simulink library "tp333079"  (Simulink 5.0)
values from neighbouring files (symbols this model uses):
  b = 1    [main_flock3.m]    (also in main_flock4.m; params_flocking_ros.m)
undefined symbols (not defined in the file or in its folder): AC, AlphaBnd, BetaBnd, CDda, CDde, CDdf, CDdr, CDM, CDmin, CGempty, CGgross, CL0, CLa, CLalphadot, Clbeta, Clda, CLde, CLdf, Cldr, CLM, CLmind, Clp, CLq, Clr, Cm0, Cma, Cmalphadot, Cmde, Cmdf, CmM, Cmq, Cnbeta, Cnda, Cndr, Cnp, Cnr, CP, CT, CYbeta, CYda, CYdr, CYp, CYr, Displacement, dmy, Engine, EulerIni, FuelFlow, FuelIni, J, Jempty, Jeng, Jgross, Jprop, MAC, MAP, MAPLim, MassIni, MaxPower, mempty ... (+26)
libraries: aerosimlib x325, simulink3 x42
(part 2 of 11)

== system tp333079/Inertia ==
  Aircraft Inertia : Subsystem  SimViewingDevice=off  mask(Aircraft inertia){FuelIni=FuelIni, Mempty=mempty, Mgross=mgross, CGempty=CGempty, CGgross=CGgross, Jempty=Jempty, Jgross=Jgross}
      mask prompts: FuelIni "Initial fuel mass:"; Mempty "Empty mass:"; Mgross "Gross mass:"; CGempty "Empty CG location [X Y Z]:"; CGgross "Gross CG location [X Y Z]:"; Jempty "Empty moments of inertia [Jx Jy Jz Jxz]:"; Jgross "Gross moments of inertia [Jx Jy Jz Jxz]:"
      mask help: Computes the current aircraft inertia parameters (mass, CG location and moments of inertia) given the fuel flow.
      settings: Permissions=ReadWrite  RTWFcnNameOpts=Auto  RTWFileNameOpts=Auto
      mask Help:
      | The block integrates the fuel flow rate and updates the inertia parameters of the airpane knowing the current fuel quantity.
      | <P><B>Parameters:</B>
      | <LI>Initial fuel mass;</LI>
      | <LI>Mass of empty aircraft;</LI>
      | <LI>Gross mass of the aircraft;</LI>
      | <LI>The 3x1 position vector from origin to the empty aircraft CG location;</LI>
      | <LI>The 3x1 position vector from origin to the gross aircraft CG location;</LI>
      | <LI>The 4x1 vector of moments of inertia for the empty aircraft;</LI>
      | <LI>The 4x1 vector of moments of inertia for the gross aircraft;</LI>
      | </P>
      | <P><B>Inputs:</B>
      | <LI>Fuel flow;</LI>
      | <LI>Reset flag, for resetting the fuel integrator back to the initial value;</LI>
      | </P>
      | <P><B>Outputs:</B>
      | <LI>Current aircraft mass;</LI>
      | <LI>Current aircraft CG location;</LI>
      | <LI>Current aircraft moments of inertia.</LI>
      | <LI>Flag that gets set to 1 if the aircraft is out of fuel.</LI>
      | </P>
  Inertia Coefficients : Subsystem  SimViewingDevice=off
      settings: Permissions=ReadWrite  RTWFcnNameOpts=Auto  RTWFileNameOpts=Auto
      mask Type: Inertia coefficients
      mask Description: Compute inertia coefficients c1-c10 based on moments of inertia.
      mask Help:
      | The block computes the coefficients c1-c10 which are elements of the inverse of the moments of inertia matrix, used in the rigid body moment equations.
      | <P><B>Input:</B> 4x1 vector of moments of inertia;</P>
      | <P><B>Output:</B> 10x1 vector of inertia coefficients.</P>

== system tp333079/Math ==
  2pi Bound : Subsystem  SimViewingDevice=off
      settings: Permissions=ReadWrite  RTWFcnNameOpts=Auto  RTWFileNameOpts=Auto
      mask Type: 2pi bound
      mask Description: Bounds the input angle to [0, 2pi]. When 0 bound is exceeded the output wraps back to 2pi; when the 2pi bound is exceeded the output wraps back to 0.
      mask Help:
      | Bounds the input angle to [0, 2pi]. When 0 bound is exceeded the output wraps back to 2pi; when the 2pi bound is exceeded the output wraps back to 0.
      | <P><B>Input:</B> any angle in radians, from -Inf to Inf;</P>
      | <P><B>Output:</B> an angle in radians between zero and 2pi.</P>
  Cross Product : Subsystem  SimViewingDevice=off
      settings: Permissions=ReadWrite  RTWFcnNameOpts=Auto  RTWFileNameOpts=Auto
      mask Type: Cross product
      mask Description: Computes the cross product of two vectors.
      mask Help:
      | The block computes the cross product of two three-dimensional vectors.
      | <P><B>Inputs:</B> two 3x1 vectors;</P>
      | <P><B>Output:</B> the 3x1 cross product vector.</P>
  Non-zero Sign : Subsystem  SimViewingDevice=off
      settings: Permissions=ReadWrite  RTWFcnNameOpts=Auto  RTWFileNameOpts=Auto
      mask Type: Non-zero sign
      mask Description: Sign function outputs 1 for input greater than or equal to 0, and -1 otherwise.
      mask Help: Sign function outputs 1 for input greater than or equal to 0, and -1 otherwise.
  Normalization : Subsystem  SimViewingDevice=off
      settings: Permissions=ReadWrite  RTWFcnNameOpts=Auto  RTWFileNameOpts=Auto
      mask Type: Vector normalization
      mask Description: Normalize a vector, e = v/|v|.
      mask Help:
      | The block normalizes the input vector.
      | <P><B>Input:</B> the nx1 vector;</P>
      | <P><B>Output:</B> the nx1 unit vector.</P>
  Vector norm : Subsystem  SimViewingDevice=off
      settings: Permissions=ReadWrite  RTWFcnNameOpts=Auto  RTWFileNameOpts=Auto
      mask Type: Vector norm-2
      mask Description: Compute the 2-norm (magnitude) of a vector, |v| = sqrt(v'v).
      mask Help:
      | The block compute the 2-norm (or magnitude) of a vector.
      | <P><B>Input:</B> nx1 vector;</P>
      | <P><B>Output:</B> scalar magnitude.</P>
  Zero Offset : Subsystem  SimViewingDevice=off  mask(Zero offset){tol=10^-6}
      mask prompts: tol "Tolerance"
      mask help: This block outputs a value equal to the tolerance specified in the block parameters if the input falls within a sphere with this tolerance as radius and center in the origin. Otherwise, the output equals the input.
      settings: Permissions=ReadWrite  RTWFcnNameOpts=Auto  RTWFileNameOpts=Auto
      mask Help: This block outputs a value equal to the tolerance specified in the block parameters if the input falls within a sphere with this tolerance as radius and center in the origin. Otherwise, the output equals the input.
  pi Bound : Subsystem  SimViewingDevice=off
      settings: Permissions=ReadWrite  RTWFcnNameOpts=Auto  RTWFileNameOpts=Auto
      mask Type: pi bound
      mask Description: Bounds the input angle to [-pi, pi]. When -pi bound is exceeded the output wraps back to pi; when the pi bound is exceeded the output wraps back to -pi.
      mask Help:
      | Bounds the input angle to [-pi, pi]. When -pi bound is exceeded the output wraps back to pi; when the pi bound is exceeded the output wraps back to -pi.
      | <P><B>Input:</B> any angle in radians, from -Inf to Inf;</P>
      | <P><B>Output:</B> an angle in radians between -pi and pi.</P>

== system tp333079/Pilot Interface ==
  CH F-16 Combat Stick : Subsystem  SimViewingDevice=off  mask(CH F-16 Combat Stick){tsamp=0.02}
      mask prompts: tsamp "Sample time:"
      mask help: Joystick interface for F-16 Combat Stick by CH Products.
      settings: Permissions=ReadWrite  RTWFcnNameOpts=Auto  RTWFileNameOpts=Auto
      mask Help:
      | The block provides interface for the F-16 Combat Stick by CH Products.
      | <P><B>Outputs:</B>
      | <LI>Horiz axis = the current joystick position on the horizontal axis</LI>
      | <LI>Vert axis = the current joystick position on the vertical axis</LI>
      | <LI>Throttle axis = the current position of the throttle wheel</LI>
      | <LI>POV = the current state of the joystick hat switch (0=center, 1=up, -1=down, 2=right, -2=left)</LI>
      | <LI>Button 1-9 = the current states of the 9 available buttons</LI>
      | </P>
      | <P><B>Parameters:</B>
      | <LI>Sample time = the time interval at which the joystick data is sampled</LI>
      | </P>
  FS Interface : Subsystem  SimViewingDevice=off  mask(FS interface){tsamp=0.2}
      mask prompts: tsamp "Sample time:"
      mask help: Microsoft Flight Simulator Interface that provides a visual output of the aircraft position and attitude.
      settings: Permissions=ReadWrite  RTWFcnNameOpts=Auto  RTWFileNameOpts=Auto
      mask Help:
      | The block provides position and attitude information to Microsoft Flight Simulator for visual output of the aircraft behavior. The data transfer is based on Inter-Process Communication using FSUIPC module.
      | <P><B>Inputs:</B>
      | <LI> the 3x1 vector of geographic position;</LI>
      | <LI> the 3x1 vector of Euler angles;</LI>
      | <LI> scalar number representing airspeed.</LI></P>
  FlightGear Interface : Subsystem  SimViewingDevice=off  mask(FlightGear interface){hostname='localhost', tsamp=0.2}
      mask prompts: hostname "Host name:"; tsamp "Sample time:"
      mask help: FlightGear Flight Simulator Interface that provides a visual output of the aircraft position and attitude.
      settings: Permissions=ReadWrite  RTWFcnNameOpts=Auto  RTWFileNameOpts=Auto
      mask Help:
      | The block provides position and attitude information to FlightGear Flight Simulator for visual output of the aircraft behavior.
      | <P><B>Parameters:</B>
      | <LI>Sample time: the sample time at which data is sent to FlightGear;</LI>
      | <LI>Host name: the name or IP address of the machine on which FlightGear is running.</LI></P>
      | <P><B>Inputs:</B>
      | <LI> the 3x1 vector of geographic position;</LI>
      | <LI> the 3x1 vector of Euler angles;</LI>
      | <LI> scalar number representing airspeed.</LI></P>
  Joystick Interface : Subsystem  SimViewingDevice=off  mask(Joystick interface){tsamp=0.02}
      mask prompts: tsamp "Sample time:"
      mask help: Generic Windows joystick interface.
      settings: Permissions=ReadWrite  RTWFcnNameOpts=Auto  RTWFileNameOpts=Auto
      mask Help:
      | The block provides a generic Windows joystick interface.
      | <P><B>Outputs:</B>
      | <LI>Axes = the 6x1 vector of current joystick position on the 6 available axes</LI>
      | <LI>Buttons = the 32x1 vector of current states of the 32 available buttons (0 or 1)</LI>
      | <LI>POV = the current state of the joystick hat switch (0=center, 1=up, -1=down, 2=right, -2=left)</LI>
      | </P>
      | <P><B>Parameters:</B>
      | <LI>Sample time = the time interval at which the joystick data is sampled</LI>
      | </P>

== system tp333079/Propulsion ==
  Fixed-pitch Propeller : Subsystem  SimViewingDevice=off  mask(Fixed-pitch propeller model){J=J, CT=CT, CP=CP, R=Rprop}
      mask prompts: J "Advance ratio:"; CT "Coefficient of thrust:"; CP "Coefficient of power:"; R "Radius:"
      mask help: Fixed-pitch propeller model using look-up tables of thrust and power coefficients as functions of advance ratio.
      settings: Permissions=ReadWrite  RTWFcnNameOpts=Auto  RTWFileNameOpts=Auto
      mask Help:
      | The block provides a fixed-pitch propeller model based on look-up tables for thrust and power coefficients as function of the advance ratio.
      | <P><B>Inputs:</B>
      | <LI>Airspeed = the current aircraft airspeed</LI>
      | <LI>rho = the air density at current aircraft altitude</LI>
      | <LI>Omega = the propeller rotation speed</LI>
      | </P>
      | <P><B>Output:</B>
      | <LI>Fprop = the thrust force generated by the propeller (on body x-axis)</LI>
      | <LI>Mprop = the moment generated by the propeller (on body x-axis)</LI>
      | <LI>PropCoeff = the 3x1 vector of propeller coefficients [J CT CP]</LI>
      | </P>
      | <P><B>Parameters:</B>
      | <LI>Advance ratio = the advance ratio vector for interpolation</LI>
      | <LI>Coefficient of thrust = the coefficient of thrust vector for interpolation</LI>
      | <LI>Coefficient of power = the coefficient of power vector for interpolation</LI>
      | <LI>Radius = the propeller radius</LI>
      | </P>
  GA Propulsion System : Subsystem  SimViewingDevice=off  mask(General-aviation propulsion system){OmegaIni=OmegaIni, RPM=RPM, MAP=MAP, FuelFlow=FuelFlow, Power=Power, Jeng=Jeng, J=J, CT=CT, CP=CP, Rprop=Rprop, Jprop=Jprop, TSL=TSL}
      mask prompts: OmegaIni "Initial engine speed:"; RPM "Engine RPM vector:"; MAP "Engine MAP vector:"; FuelFlow "Engine fuel flow look-up table:"; Power "Engine power look-up table:"; Jeng "Engine moment of inertia:"; J "Propeller advance ratio vector:"; CT "Propeller coefficient of thrust vector:"; CP "Propeller coefficient of power vector:"; Rprop "Propeller radius:"; Jprop "Propeller moment of inertia:"; TSL "Sea-level temperature:"
      mask help: The block models a general aviation propulsion system including a piston engine and a fixed-pitch propeller.
      settings: Permissions=ReadWrite  RTWFcnNameOpts=Auto  RTWFileNameOpts=Auto
      mask Help:
      | The block provides a general aviation propulsion system using the AeroSim piston engine and fixed-pitch propeller models.
      | <P><B>Inputs:</B>
      | <LI>Control = the 3x1 engine control vector [Throttle Mixture Ignition]</LI>
      | <LI>OutofFuel = the out-of-fuel flag (0 or 1)</LI>
      | <LI>p = the static pressure at current altitude, in Pa</LI>
      | <LI>T = the air temperature at current altitude, in K</LI>
      | <LI>rho = the air density at current altitude, in kg/m^3</LI>
      | <LI>WindAxesVel = the 3x1 vector of body velocities in wind axes [Airspeed Sideslip Angle-of-attack] in [m/s rad rad]</LI>
      | <LI>RST = the integrator reset flag (rising edge)</LI>
      | </P>
      | <P><B>Output:</B>
      | <LI>Fprop = the 3x1 vector of propulsion system forces applied to the airframe, at the propeller hub location</LI>
      | <LI>Mprop = the 3x1 vector of propulsion system moments applied to the airframe</LI>
      | <LI>Omega = the engine shaft rotation speed, in rad/s</LI>
      | <LI>FuelFlow = the mass fuel flow, in kg/s</LI>
      | <LI>EngCoeff = the 5x1 engine coefficient vector [MAP Airflow Fuelflow BSFC Power] in [kPa kg/s kg/s g/(W*hr) W]</LI>
      | <LI>PropCoeff = the 3x1 propeller coefficient vector [J CT CP]</LI>
      | </P>
      | <P><B>Parameters:</B>
      | <LI>Initial engine speed = the initial value for the engine speed, in rad/s</LI>
      | <LI>RPM vector = the engine speed interpolation vector, in rpm</LI>
      | <LI>MAP vector = the manifold air pressure interpolation vector, in kPa</LI>
      | <LI>Fuel flow = the 2-D look-up table for fuel flow, as function of MAP and RPM, in g/hr</LI>
      | <LI>Power = the 2-D look-up table for power, as function of MAP and RPM, in W</LI>
      | <LI>Engine moment of inertia = the moment of inertia of the rotating engine parts (shaft)</LI>
      | <LI>Advance ratio = the advance ratio vector for interpolation</LI>
      | <LI>Coefficient of thrust = the coefficient of thrust vector for interpolation</LI>
      | <LI>Coefficient of power = the coefficient of power vector for interpolation</LI>
      | <LI>Radius = the propeller radius</LI>
      | <LI>Propeller moment of inertia = the moment of inertia of the propeller</LI>
      | <LI>Sea-level temperature = the ambient temperature for which the above engine look-up tables are given</LI>
      | </P>
  Piston Engine : Subsystem  SimViewingDevice=off  mask(Piston Engine){RPM=RPM, MAP=MAP, fflow=FuelFlow, Power=Power, TSL=TSL}
      mask prompts: RPM "RPM vector:"; MAP "MAP vector:"; fflow "Fuel flow 2-D look-up table:"; Power "Power 2-D look-up table:"; TSL "Sea-level temperature:"
      mask help: The piston engine model computes the engine parameters at current throttle setting, engine rpm, and altitude.
      settings: Permissions=ReadWrite  RTWFcnNameOpts=Auto  RTWFileNameOpts=Auto
      mask Help:
      | The block provides a piston engine model based on look-up tables for manifold pressure, engine speed (rpm), fuel flow and power.
      | <P><B>Inputs:</B>
      | <LI>Thr = the throttle command (as a fraction of atmospheric pressure)</LI>
      | <LI>Mix = the air to fuel mixture ratio</LI>
      | <LI>Omega = the engine shaft rotation speed</LI>
      | <LI>p = the atmospheric pressure, in Pa</LI>
      | <LI>T = the atmospheric temperature, in K</LI>
      | </P>
      | <P><B>Output:</B>
      | <LI>MAP = the manifold air pressure, in kPa</LI>
      | <LI>AirFlow = the mass air flow, in kg/s</LI>
      | <LI>FuelFlow = the mass fuel flow, in kg/s</LI>
      | <LI>BSFC = the brake-specific fuel consumption, in g/(W*hr)</LI>
      | <LI>Power = the engine power, in W</LI>
      | <LI>Torque = the engine shaft torque, in N*m</LI>
      | </P>
      | <P><B>Parameters:</B>
      | <LI>RPM vector = the engine speed interpolation vector, in rpm</LI>
      | <LI>MAP vector = the manifold air pressure interpolation vector, in kPa</LI>
      | <LI>Fuel flow = the 2-D look-up table for fuel flow, as function of MAP and RPM, in g/hr</LI>
      | <LI>Power = the 2-D look-up table for power, as function of MAP and RPM, in W</LI>
      | <LI>Sea-level temperature = the ambient temperature for which the above engine look-up tables are given</LI>
      | </P>

== system tp333079/Sensors ==
  Analog Sensors : Subsystem  SimViewingDevice=off
      settings: Permissions=ReadWrite  RTWFcnNameOpts=Auto  RTWFileNameOpts=Auto
  Digital Sensors : Subsystem  SimViewingDevice=off
      settings: Permissions=ReadWrite  RTWFcnNameOpts=Auto  RTWFileNameOpts=Auto
  Generic Sensors : Subsystem  SimViewingDevice=off
      settings: Permissions=ReadWrite  RTWFcnNameOpts=Auto  RTWFileNameOpts=Auto
  Noise Correlation : Subsystem  SimViewingDevice=off
      settings: Permissions=ReadWrite  RTWFcnNameOpts=Auto  RTWFileNameOpts=Auto

== system tp333079/Transformations ==
  Body-Inertial DCM From Euler Angles : Subsystem  SimViewingDevice=off
      settings: Permissions=ReadWrite  RTWFcnNameOpts=Auto  RTWFileNameOpts=Auto
      mask Type: Body-Inertial DCM
      mask Description: Compute the direction cosine matrix required for inertial-to-body frame transformation.
      mask Help:
      | The block computes the Direction Cosine matrix which is the rotation matrix from inertial to body frame, given the vehicle attitude in Euler angles.
      | <P><B>Input:</B> the 3x1 vector of Euler angles;</P>
      | <P><B>Output:</B> the 3x3 Direction Cosine matrix.</P>
  Body-Inertial DCM From Quaternions : Subsystem  SimViewingDevice=off
      settings: Permissions=ReadWrite  RTWFcnNameOpts=Auto  RTWFileNameOpts=Auto
      mask Type: Body-Inertial DCM
      mask Description: Compute the direction cosine matrix required for inertial-to-body frame transformation.
      mask Help:
      | The block computes the Direction Cosine matrix which is the rotation matrix from inertial to body frame, given the Euler-Rodrigues quaternions.
      | <P><B>Input:</B> the 4x1 vector of quaterions;</P>
      | <P><B>Output:</B> the 3x3 Direction Cosine matrix.</P>
  Body-Wind DCM : Subsystem  SimViewingDevice=off
      settings: Permissions=ReadWrite  RTWFcnNameOpts=Auto  RTWFileNameOpts=Auto
      mask Type: Body-Wind DCM
      mask Description: Compute the body-axes to wind-axes direction cosine matrix.
      mask Help:
      | The block computes the Direction Cosine matrix that defines the rotation from body to wind axes, given the sideslip angle and the angle-of-attack.
      | <P><B>Input:</B> the 3x1 vector of wind axes velocity components (airspeed, sideslip, angle-of-attack);</P>
      | <P><B>Output:</B> the 3x3 Direction Cosine matrix.</P>
  ECEF Position : Subsystem  SimViewingDevice=off
      settings: Permissions=ReadWrite  RTWFcnNameOpts=Auto  RTWFileNameOpts=Auto
      mask Type: ECEF Position
      mask Description: Compute ECEF (Earth-centered Earth-fixed) position from LLA (Latitude, Longitude, Altitude) position.
      mask Help:
      | The block computes the coordinates of the vehicle in the Earth-Centered Earth-Fixed frame, given the coordinates in geographic frame and local Earth radii.
      | <P><B>Inputs:</B>
      | <LI>LLA = the 3x1 position vector (Latitude, Longitude, Altitude);</LI>
      | <LI>Rmeridian = local meridian radius of the Earth;</LI>
      | <LI>Rnormal = local normal radius of the Earth;</LI></P>
      | <P><B>Output:</B> the 3x1 vector of ECEF position (X, Y, Z).</P>
  Euler Angles From Quaternions : Subsystem  SimViewingDevice=off
      settings: Permissions=ReadWrite  RTWFcnNameOpts=Auto  RTWFileNameOpts=Auto
      mask Type: Euler Angles
      mask Description: Compute Euler angles from Euler-Rodrigues quaternions.
      mask Help:
      | The block computes the three Euler angles (roll, pitch, heading) of the vehicle based on the Euler-Rodrigues quaternions.
      | <P><B>Input:</B> the 4x1 vector of quaternions;</P>
      | <P><B>Output:</B> the 3x1 vector of Euler angles.</P>
  Euler Angles  From DCM : Subsystem  SimViewingDevice=off
      settings: Permissions=ReadWrite  RTWFcnNameOpts=Auto  RTWFileNameOpts=Auto
      mask Type: Euler angles from DCM
      mask Description: Compute Euler angles given the Direction Cosine Matrix.
      mask Help:
      | The block extracts the 3 Euler angles (roll, pitch, and heading) from elements of the Direction Cosine matrix.
      | <P><B>Input:</B> a 3x3 Direction Cosine matrix;</P>
      | <P><B>Output:</B> a 3x1 vector with the Euler angles.</P>
  Quaternions From Euler Angles : Subsystem  SimViewingDevice=off
      settings: Permissions=ReadWrite  RTWFcnNameOpts=Auto  RTWFileNameOpts=Auto
      mask Type: Quaternions
      mask Description: Compute quaternions from Euler angles.
      mask Help:
      | The block computes the four quaternions (q0, qx, qy, qz) of the vehicle based on the Euler angles.
      | <P><B>Input:</B> the 3x1 vector of Euler angles.</P>
      | <P><B>Output:</B> the 4x1 vector of quaternions;</P>

== system tp333079/Unit Conversion ==
  Angular position : Subsystem  SimViewingDevice=off
      settings: Permissions=ReadWrite  RTWFcnNameOpts=Auto  RTWFileNameOpts=Auto
  Angular velocity : Subsystem  SimViewingDevice=off
      settings: Permissions=ReadWrite  RTWFcnNameOpts=Auto  RTWFileNameOpts=Auto
  Distance : Subsystem  SimViewingDevice=off
      settings: Permissions=ReadWrite  RTWFcnNameOpts=Auto  RTWFileNameOpts=Auto
  Force : Subsystem  SimViewingDevice=off
      settings: Permissions=ReadWrite  RTWFcnNameOpts=Auto  RTWFileNameOpts=Auto
  Mass : Subsystem  SimViewingDevice=off
      settings: Permissions=ReadWrite  RTWFcnNameOpts=Auto  RTWFileNameOpts=Auto
  Pressure : Subsystem  SimViewingDevice=off
      settings: Permissions=ReadWrite  RTWFcnNameOpts=Auto  RTWFileNameOpts=Auto
  Temperature : Subsystem  SimViewingDevice=off
      settings: Permissions=ReadWrite  RTWFcnNameOpts=Auto  RTWFileNameOpts=Auto
  Velocity : Subsystem  SimViewingDevice=off
      settings: Permissions=ReadWrite  RTWFcnNameOpts=Auto  RTWFileNameOpts=Auto
  Volume : Subsystem  SimViewingDevice=off
      settings: Permissions=ReadWrite  RTWFcnNameOpts=Auto  RTWFileNameOpts=Auto

== system tp333079/Actuators/D/A Converter ==
  Digital : Inport  Port=1  PortDimensions=-1  SampleTime=-1  DataType=auto
      settings: SignalType=auto
  Count size in Volts : Product  Inputs=*/  Multiplication=Element-wise(.*)  SaturateOnIntegerOverflow=on
  Max Counts : Constant  Value=2^Bits
  Max Volts : Constant  Value=MaxVolts
  Min Volts : Constant  Value=MinVolts
  Saturation : Saturate  UpperLimit=MaxVolts  LowerLimit=MinVolts  LinearizeAsGain=on
  Sum : Sum  Inputs=|+-  SaturateOnIntegerOverflow=on
  Voltage : Product  Inputs=2  Multiplication=Element-wise(.*)  SaturateOnIntegerOverflow=on
  Analog : Outport  Port=1
  wires:
  Digital/1 -> Voltage/1
  Voltage/1 -> Saturation/1
  Max Volts/1 -> Sum/1
  Min Volts/1 -> Sum/2
  Max Counts/1 -> Count size in Volts/2
  Sum/1 -> Count size in Volts/1
  Count size in Volts/1 -> Voltage/2
  Saturation/1 -> Analog/1

== system tp333079/Actuators/Simple Actuator (1st-order dynamics) ==
  Input : Inport  Port=1  PortDimensions=1  SampleTime=-1  DataType=auto
      settings: SignalType=auto
  Look-Up Table : Lookup  InputValues=[MinCounts MaxCounts]  OutputValues=[MinAct MaxAct]
  Rate Limiter : RateLimiter  RisingSlewLimit=MaxRate  FallingSlewLimit=-MaxRate
  Saturation : Saturate  UpperLimit=MaxCounts  LowerLimit=MinCounts  LinearizeAsGain=on
  Transfer Fcn : TransferFcn  Numerator=[1]  Denominator=[Lag 1]  AbsoluteTolerance=auto  Realization=auto
  Output : Outport  Port=1
  wires:
  Transfer Fcn/1 -> Output/1
  Rate Limiter/1 -> Transfer Fcn/1
  Saturation/1 -> Look-Up Table/1
  Input/1 -> Saturation/1
  Look-Up Table/1 -> Rate Limiter/1

== system tp333079/Actuators/Simple Actuator (2nd-order dynamics) ==
  Input : Inport  Port=1  PortDimensions=1  SampleTime=-1  DataType=auto
      settings: SignalType=auto
  Look-Up Table : Lookup  InputValues=[MinCounts MaxCounts]  OutputValues=[MinAct MaxAct]
  Rate Limiter : RateLimiter  RisingSlewLimit=MaxRate  FallingSlewLimit=-MaxRate
  Saturation : Saturate  UpperLimit=MaxCounts  LowerLimit=MinCounts  LinearizeAsGain=on
  Transfer Fcn : TransferFcn  Numerator=[wn^2]  Denominator=[1 2*zeta*wn wn^2]  AbsoluteTolerance=auto  Realization=auto
  Output : Outport  Port=1
  wires:
  Look-Up Table/1 -> Rate Limiter/1
  Input/1 -> Saturation/1
  Saturation/1 -> Look-Up Table/1
  Rate Limiter/1 -> Transfer Fcn/1
  Transfer Fcn/1 -> Output/1

== system tp333079/Aerodynamics/Aerodynamic Force ==
  note: Get aerodynamic forces in
      | wind axes
  note: Get aerodynamic forces
      | in body axes
  CD : Inport  Port=1  PortDimensions=1  SampleTime=-1  DataType=auto
      settings: SignalType=auto
  CY : Inport  Port=2  PortDimensions=1  SampleTime=-1  DataType=auto
      settings: SignalType=auto
  CL : Inport  Port=3  PortDimensions=1  SampleTime=-1  DataType=auto
      settings: SignalType=auto
  pdyn : Inport  Port=4  PortDimensions=1  SampleTime=-1  DataType=auto
      settings: SignalType=auto
  WindAxesVel : Inport  Port=5  PortDimensions=[3 1]  SampleTime=-1  DataType=auto
      settings: SignalType=auto
  Body-Wind DCM : aerosimlib/Transformations/Body-Wind DCM
  ChSign : Gain  Gain=-1  Multiplication=Element-wise(K.*u)  SaturateOnIntegerOverflow=on
  ChSign1 : Gain  Gain=-1  Multiplication=Element-wise(K.*u)  SaturateOnIntegerOverflow=on
  DCM' : Math  Operator=transpose  OutputSignalType=auto
  Mux : Mux  Inputs=3
  Product : Product  Inputs=3  Multiplication=Element-wise(.*)  SaturateOnIntegerOverflow=on
  Product1 : Product  Inputs=2  Multiplication=Matrix(*)  SaturateOnIntegerOverflow=on
  Wing area : Constant  Value=S
  Faero : Outport  Port=1
  wires:
  ChSign1/1 -> Mux/3
  ChSign/1 -> Mux/1
  CD/1 -> ChSign/1
  CY/1 -> Mux/2
  CL/1 -> ChSign1/1
  Mux/1 -> Product/1
  pdyn/1 -> Product/2
  Wing area/1 -> Product/3
  WindAxesVel/1 -> Body-Wind DCM/1
  DCM'/1 -> Product1/1
  Body-Wind DCM/1 -> DCM'/1
  Product/1 -> Product1/2
  Product1/1 -> Faero/1

== system tp333079/Aerodynamics/Aerodynamic Moment ==
  note: Sources
  note: Compute moments
  note: Output
  Cl : Inport  Port=1  PortDimensions=1  SampleTime=-1  DataType=auto
      settings: SignalType=auto
  Cm : Inport  Port=2  PortDimensions=1  SampleTime=-1  DataType=auto
      settings: SignalType=auto
  Cn : Inport  Port=3  PortDimensions=1  SampleTime=-1  DataType=auto
      settings: SignalType=auto
  pdyn : Inport  Port=4  PortDimensions=1  SampleTime=-1  DataType=auto
      settings: SignalType=auto
  Mux : Mux  Inputs=3
  Pitch : Product  Inputs=4  Multiplication=Element-wise(.*)  SaturateOnIntegerOverflow=on
  Roll : Product  Inputs=4  Multiplication=Element-wise(.*)  SaturateOnIntegerOverflow=on
  Wing area : Constant  Value=S
  Wing chord : Constant  Value=c
  Wing span : Constant  Value=b
  Yaw : Product  Inputs=4  Multiplication=Element-wise(.*)  SaturateOnIntegerOverflow=on
  Maero : Outport  Port=1
  wires:
  Cl/1 -> Roll/4
  Cm/1 -> Pitch/4
  Cn/1 -> Yaw/4
  pdyn/1 -> Roll/1, Pitch/1, Yaw/1
  Wing area/1 -> Roll/2, Pitch/2, Yaw/2
  Wing chord/1 -> Pitch/3
  Wing span/1 -> Roll/3, Yaw/3
  Roll/1 -> Mux/1
  Mux/1 -> Maero/1
  Pitch/1 -> Mux/2
  Yaw/1 -> Mux/3

== system tp333079/Aerodynamics/Drag Coefficient ==
  note: Drag component build-up
  note: Sources
  WindAxesVel : Inport  Port=1  PortDimensions=[3 1]  SampleTime=-1  DataType=auto
      settings: SignalType=auto
  Control : Inport  Port=2  PortDimensions=[4 1]  SampleTime=-1  DataType=auto
      settings: SignalType=auto
  CL : Inport  Port=3  PortDimensions=1  SampleTime=-1  DataType=auto
      settings: SignalType=auto
  Mach : Inport  Port=4  PortDimensions=1  SampleTime=-1  DataType=auto
      settings: SignalType=auto
  Abs{,1..3} (4 alike) : Abs  SaturateOnIntegerOverflow=on
  CD0 : Constant  Value=CD0
  CDM : Gain  Gain=CDM  Multiplication=Element-wise(K.*u)  SaturateOnIntegerOverflow=on
  CDda : Gain  Gain=CDda  Multiplication=Element-wise(K.*u)  SaturateOnIntegerOverflow=on
  CDde : Gain  Gain=CDde  Multiplication=Element-wise(K.*u)  SaturateOnIntegerOverflow=on
  CDdf : Gain  Gain=CDdf  Multiplication=Element-wise(K.*u)  SaturateOnIntegerOverflow=on
  CDdr : Gain  Gain=CDdr  Multiplication=Element-wise(K.*u)  SaturateOnIntegerOverflow=on
  CL min drag : Constant  Value=CL0
  CL^2 : Math  Operator=square  OutputSignalType=auto
  Demux : Demux  Outputs=4  BusSelectionMode=off
  Demux1 : Demux  Outputs=3  BusSelectionMode=off
  Induced Drag : Gain  Gain=k  Multiplication=Element-wise(K.*u)  SaturateOnIntegerOverflow=on
  Sum : Sum  Inputs=|+-  SaturateOnIntegerOverflow=on
  Sum2 : Sum  Inputs=+++++++  SaturateOnIntegerOverflow=on
  Terminator : Terminator
  Terminator1 : Terminator
  Terminator2 : Terminator
  CD : Outport  Port=1
  wires:
  CDM/1 -> Sum2/7
  Mach/1 -> CDM/1
  CL min drag/1 -> Sum/2
  CL/1 -> Sum/1
  Sum/1 -> CL^2/1
  Sum2/1 -> CD/1
  CDdr/1 -> Abs3/1
  CDda/1 -> Abs2/1
  CDde/1 -> Abs1/1
  CDdf/1 -> Abs/1
  Induced Drag/1 -> Sum2/2
  CD0/1 -> Sum2/1
  CL^2/1 -> Induced Drag/1
  Control/1 -> Demux/1
  Demux/4 -> CDdr/1
  Demux/3 -> CDda/1
  Demux/2 -> CDde/1
  Demux/1 -> CDdf/1
  WindAxesVel/1 -> Demux1/1
  Abs/1 -> Sum2/3
  Abs1/1 -> Sum2/4
  Abs2/1 -> Sum2/5
  Abs3/1 -> Sum2/6
  Demux1/1 -> Terminator/1
  Demux1/2 -> Terminator1/1
  Demux1/3 -> Terminator2/1

== system tp333079/Aerodynamics/Dynamic Pressure ==
  WindAxesVel : Inport  Port=1  PortDimensions=[3 1]  SampleTime=-1  DataType=auto
      settings: SignalType=auto
  rho : Inport  Port=2  PortDimensions=1  SampleTime=-1  DataType=auto
      settings: SignalType=auto
  0.5*rho*Va^2 : Product  Inputs=2  Multiplication=Element-wise(.*)  SaturateOnIntegerOverflow=on
  Demux : Demux  Outputs=3  BusSelectionMode=off
  Gain : Gain  Gain=1/2  Multiplication=Element-wise(K.*u)  SaturateOnIntegerOverflow=on
  Terminator : Terminator
  Terminator1 : Terminator
  Va^2 : Math  Operator=square  OutputSignalType=auto
  pdyn : Outport  Port=1
  wires:
  rho/1 -> Gain/1
  Demux/3 -> Terminator1/1
  Demux/2 -> Terminator/1
  Demux/1 -> Va^2/1
  WindAxesVel/1 -> Demux/1
  Va^2/1 -> 0.5*rho*Va^2/1
  Gain/1 -> 0.5*rho*Va^2/2
  0.5*rho*Va^2/1 -> pdyn/1

== system tp333079/Aerodynamics/Lift Coefficient ==
  note: Lift component build-up
  note: Sources
  WindAxesVel : Inport  Port=1  PortDimensions=[3 1]  SampleTime=-1  DataType=auto
      settings: SignalType=auto
  Control : Inport  Port=2  PortDimensions=[4 1]  SampleTime=-1  DataType=auto
      settings: SignalType=auto
  AlphaBetaDot : Inport  Port=3  PortDimensions=[2 1]  SampleTime=-1  DataType=auto
      settings: SignalType=auto
  AngularRates : Inport  Port=4  PortDimensions=[3 1]  SampleTime=-1  DataType=auto
      settings: SignalType=auto
  Mach : Inport  Port=5  PortDimensions=1  SampleTime=-1  DataType=auto
      settings: SignalType=auto
  2 : Gain  Gain=2  Multiplication=Element-wise(K.*u)  SaturateOnIntegerOverflow=on
  CL*c/(2V) : Product  Inputs=**/  Multiplication=Element-wise(.*)  SaturateOnIntegerOverflow=on
  CL0 : Constant  Value=CL0
  CLM : Gain  Gain=CLM  Multiplication=Element-wise(K.*u)  SaturateOnIntegerOverflow=on
  CLalpha : Gain  Gain=CLalpha  Multiplication=Element-wise(K.*u)  SaturateOnIntegerOverflow=on
  CLalphadot : Gain  Gain=CLalphadot  Multiplication=Element-wise(K.*u)  SaturateOnIntegerOverflow=on
  CLde : Gain  Gain=CLde  Multiplication=Element-wise(K.*u)  SaturateOnIntegerOverflow=on
  CLdf : Gain  Gain=CLdf  Multiplication=Element-wise(K.*u)  SaturateOnIntegerOverflow=on
  CLq : Gain  Gain=CLq  Multiplication=Element-wise(K.*u)  SaturateOnIntegerOverflow=on
  Demux : Demux  Outputs=4  BusSelectionMode=off
  Demux1 : Demux  Outputs=3  BusSelectionMode=off
  Demux2 : Demux  Outputs=2  BusSelectionMode=off
  Demux3 : Demux  Outputs=3  BusSelectionMode=off
  Sum : Sum  Inputs=++  SaturateOnIntegerOverflow=on
  Sum2 : Sum  Inputs=++++++  SaturateOnIntegerOverflow=on
  Terminator{,1..5} (6 alike) : Terminator
  Wing chord : Constant  Value=c
  CL : Outport  Port=1
  wires:
  CLM/1 -> Sum2/6
  Mach/1 -> CLM/1
  Demux3/3 -> Terminator5/1
  Demux3/2 -> CLq/1
  Demux3/1 -> Terminator4/1
  AngularRates/1 -> Demux3/1
  Sum2/1 -> CL/1
  CL*c/(2V)/1 -> Sum2/5
  CLde/1 -> Sum2/4
  CLdf/1 -> Sum2/3
  CLalpha/1 -> Sum2/2
  CL0/1 -> Sum2/1
  Sum/1 -> CL*c/(2V)/1
  CLalphadot/1 -> Sum/1
  AlphaBetaDot/1 -> Demux2/1
  Demux2/2 -> Terminator3/1
  Demux2/1 -> CLalphadot/1
  Control/1 -> Demux/1
  Demux/4 -> Terminator2/1
  Demux/3 -> Terminator1/1
  Demux/2 -> CLde/1
  Demux/1 -> CLdf/1
  Demux1/3 -> CLalpha/1
  Demux1/2 -> Terminator/1
  Demux1/1 -> 2/1
  CLq/1 -> Sum/2
  Wing chord/1 -> CL*c/(2V)/2
  2/1 -> CL*c/(2V)/3
  WindAxesVel/1 -> Demux1/1

== system tp333079/Aerodynamics/Pitch Moment Coefficient ==
  note: Pitch moment component build-up
  note: Sources
  WindAxesVel : Inport  Port=1  PortDimensions=[3 1]  SampleTime=-1  DataType=auto
      settings: SignalType=auto
  Control : Inport  Port=2  PortDimensions=[4 1]  SampleTime=-1  DataType=auto
      settings: SignalType=auto
  AlphaBetaDot : Inport  Port=3  PortDimensions=[2 1]  SampleTime=-1  DataType=auto
      settings: SignalType=auto
  AngularRates : Inport  Port=4  PortDimensions=[3 1]  SampleTime=-1  DataType=auto
      settings: SignalType=auto
  Mach : Inport  Port=5  PortDimensions=1  SampleTime=-1  DataType=auto
      settings: SignalType=auto
  2 : Gain  Gain=2  Multiplication=Element-wise(K.*u)  SaturateOnIntegerOverflow=on
  Cm*c/(2V) : Product  Inputs=**/  Multiplication=Element-wise(.*)  SaturateOnIntegerOverflow=on
  Cm0 : Constant  Value=Cm0
  CmM : Gain  Gain=CmM  Multiplication=Element-wise(K.*u)  SaturateOnIntegerOverflow=on
  Cmalpha : Gain  Gain=Cma  Multiplication=Element-wise(K.*u)  SaturateOnIntegerOverflow=on
  Cmalphadot : Gain  Gain=Cmalphadot  Multiplication=Element-wise(K.*u)  SaturateOnIntegerOverflow=on
  Cmde : Gain  Gain=Cmde  Multiplication=Element-wise(K.*u)  SaturateOnIntegerOverflow=on
  Cmdf : Gain  Gain=Cmdf  Multiplication=Element-wise(K.*u)  SaturateOnIntegerOverflow=on
  Cmq : Gain  Gain=Cmq  Multiplication=Element-wise(K.*u)  SaturateOnIntegerOverflow=on
  Demux : Demux  Outputs=4  BusSelectionMode=off
  Demux1 : Demux  Outputs=3  BusSelectionMode=off
  Demux2 : Demux  Outputs=2  BusSelectionMode=off
  Demux3 : Demux  Outputs=3  BusSelectionMode=off
  Sum : Sum  Inputs=++  SaturateOnIntegerOverflow=on
  Sum2 : Sum  Inputs=++++++  SaturateOnIntegerOverflow=on
  Terminator{,1..5} (6 alike) : Terminator
  Wing chord : Constant  Value=c
  Cm : Outport  Port=1
  wires:
  CmM/1 -> Sum2/6
  Sum2/1 -> Cm/1
  Cm*c/(2V)/1 -> Sum2/5
  Cmde/1 -> Sum2/4
  Cmdf/1 -> Sum2/3
  Cmalpha/1 -> Sum2/2
  Cm0/1 -> Sum2/1
  Sum/1 -> Cm*c/(2V)/1
  Cmalphadot/1 -> Sum/1
  Cmq/1 -> Sum/2
  Wing chord/1 -> Cm*c/(2V)/2
  2/1 -> Cm*c/(2V)/3
  Mach/1 -> CmM/1
  Demux3/3 -> Terminator5/1
  Demux3/2 -> Cmq/1
  Demux3/1 -> Terminator4/1
  AngularRates/1 -> Demux3/1
  AlphaBetaDot/1 -> Demux2/1
  Demux2/2 -> Terminator3/1
  Demux2/1 -> Cmalphadot/1
  Control/1 -> Demux/1
  Demux/4 -> Terminator2/1
  Demux/3 -> Terminator1/1
  Demux/2 -> Cmde/1
  Demux/1 -> Cmdf/1
  Demux1/3 -> Cmalpha/1
  Demux1/2 -> Terminator/1
  Demux1/1 -> 2/1
  WindAxesVel/1 -> Demux1/1

== system tp333079/Aerodynamics/Roll Moment Coefficient ==
  note: Roll moment component build-up
  note: Sources
  WindAxesVel : Inport  Port=1  PortDimensions=[3 1]  SampleTime=-1  DataType=auto
      settings: SignalType=auto
  Control : Inport  Port=2  PortDimensions=[4 1]  SampleTime=-1  DataType=auto
      settings: SignalType=auto
  AngularRates : Inport  Port=3  PortDimensions=[3 1]  SampleTime=-1  DataType=auto
      settings: SignalType=auto
  2 : Gain  Gain=2  Multiplication=Element-wise(K.*u)  SaturateOnIntegerOverflow=on
  Cl*b/(2V) : Product  Inputs=**/  Multiplication=Element-wise(.*)  SaturateOnIntegerOverflow=on
  Clbeta : Gain  Gain=Clbeta  Multiplication=Element-wise(K.*u)  SaturateOnIntegerOverflow=on
  Clda : Gain  Gain=Clda  Multiplication=Element-wise(K.*u)  SaturateOnIntegerOverflow=on
  Cldr : Gain  Gain=Cldr  Multiplication=Element-wise(K.*u)  SaturateOnIntegerOverflow=on
  Clp : Gain  Gain=Clp  Multiplication=Element-wise(K.*u)  SaturateOnIntegerOverflow=on
  Clr : Gain  Gain=Clr  Multiplication=Element-wise(K.*u)  SaturateOnIntegerOverflow=on
  Demux : Demux  Outputs=4  BusSelectionMode=off
  Demux1 : Demux  Outputs=3  BusSelectionMode=off
  Demux3 : Demux  Outputs=3  BusSelectionMode=off
  Sum : Sum  Inputs=++  SaturateOnIntegerOverflow=on
  Sum2 : Sum  Inputs=++++  SaturateOnIntegerOverflow=on
  Terminator{,1..3} (4 alike) : Terminator
  Wing span : Constant  Value=b
  Cl : Outport  Port=1
  wires:
  Sum2/1 -> Cl/1
  Cl*b/(2V)/1 -> Sum2/4
  Cldr/1 -> Sum2/3
  Clda/1 -> Sum2/2
  Clbeta/1 -> Sum2/1
  Demux3/3 -> Clr/1
  Demux3/2 -> Terminator3/1
  Demux3/1 -> Clp/1
  AngularRates/1 -> Demux3/1
  Control/1 -> Demux/1
  Demux/4 -> Cldr/1
  Demux/3 -> Clda/1
  Demux/2 -> Terminator2/1
  Demux/1 -> Terminator1/1
  Demux1/3 -> Terminator/1
  Demux1/2 -> Clbeta/1
  Demux1/1 -> 2/1
  WindAxesVel/1 -> Demux1/1
  2/1 -> Cl*b/(2V)/3
  Wing span/1 -> Cl*b/(2V)/2
  Sum/1 -> Cl*b/(2V)/1
  Clr/1 -> Sum/2
  Clp/1 -> Sum/1

== system tp333079/Aerodynamics/Side Force Coefficient ==
  note: Side force coefficient component build-up
  note: Sources
  WindAxesVel : Inport  Port=1  PortDimensions=[3 1]  SampleTime=-1  DataType=auto
      settings: SignalType=auto
  Control : Inport  Port=2  PortDimensions=[4 1]  SampleTime=-1  DataType=auto
      settings: SignalType=auto
  AngularRates : Inport  Port=3  PortDimensions=[3 1]  SampleTime=-1  DataType=auto
      settings: SignalType=auto
  2 : Gain  Gain=2  Multiplication=Element-wise(K.*u)  SaturateOnIntegerOverflow=on
  CY*b/(2V) : Product  Inputs=**/  Multiplication=Element-wise(.*)  SaturateOnIntegerOverflow=on
  CYbeta : Gain  Gain=CYbeta  Multiplication=Element-wise(K.*u)  SaturateOnIntegerOverflow=on
  CYda : Gain  Gain=CYda  Multiplication=Element-wise(K.*u)  SaturateOnIntegerOverflow=on
  CYdr : Gain  Gain=CYdr  Multiplication=Element-wise(K.*u)  SaturateOnIntegerOverflow=on
  CYp : Gain  Gain=CYp  Multiplication=Element-wise(K.*u)  SaturateOnIntegerOverflow=on
  CYr : Gain  Gain=CYr  Multiplication=Element-wise(K.*u)  SaturateOnIntegerOverflow=on
  Demux : Demux  Outputs=4  BusSelectionMode=off
  Demux1 : Demux  Outputs=3  BusSelectionMode=off
  Demux3 : Demux  Outputs=3  BusSelectionMode=off
  Sum : Sum  Inputs=++  SaturateOnIntegerOverflow=on
  Sum2 : Sum  Inputs=++++  SaturateOnIntegerOverflow=on
  Terminator{,1..3} (4 alike) : Terminator
  Wing span : Constant  Value=b
  CY : Outport  Port=1
  wires:
  Sum2/1 -> CY/1
  CY*b/(2V)/1 -> Sum2/4
  CYdr/1 -> Sum2/3
  CYda/1 -> Sum2/2
  CYbeta/1 -> Sum2/1
  Demux3/3 -> CYr/1
  Demux3/2 -> Terminator3/1
  Demux3/1 -> CYp/1
  AngularRates/1 -> Demux3/1
  Control/1 -> Demux/1
  Demux/4 -> CYdr/1
  Demux/3 -> CYda/1
  Demux/2 -> Terminator2/1
  Demux/1 -> Terminator1/1
  Demux1/3 -> Terminator/1
  Demux1/2 -> CYbeta/1
  Demux1/1 -> 2/1
  WindAxesVel/1 -> Demux1/1
  2/1 -> CY*b/(2V)/3
  Wing span/1 -> CY*b/(2V)/2
  Sum/1 -> CY*b/(2V)/1
  CYr/1 -> Sum/2
  CYp/1 -> Sum/1

== system tp333079/Aerodynamics/Wind-axes Velocities ==
  note: Sources
  note: Get airspeed
  note: Get angle-of-attack
  note: Get sideslip
  note: Output
  Vbody : Inport  Port=1  PortDimensions=[3 1]  SampleTime=-1  DataType=auto
      settings: SignalType=auto
  Wbody : Inport  Port=2  PortDimensions=[3 1]  SampleTime=-1  DataType=auto
      settings: SignalType=auto
  SoundSpd : Inport  Port=3  PortDimensions=1  SampleTime=-1  DataType=auto
      settings: SignalType=auto
  AOA Saturation : Saturate  UpperLimit=alphabnd(2)  LowerLimit=alphabnd(1)  LinearizeAsGain=on
  Airspeed Saturation : Saturate  UpperLimit=Vabnd(2)  LowerLimit=Vabnd(1)  LinearizeAsGain=on
  Demux : Demux  Outputs=3  BusSelectionMode=off
  Derivative : Derivative
  Mux : Mux  Inputs=3
  Mux1 : Mux  Inputs=2
  Sideslip Saturation : Saturate  UpperLimit=betabnd(2)  LowerLimit=betabnd(1)  LinearizeAsGain=on
  Sum : Sum  Inputs=|+-  SaturateOnIntegerOverflow=on
  Trigonometric Function : Trigonometry  Operator=atan  OutputSignalType=auto
  Trigonometric Function1 : Trigonometry  Operator=asin  OutputSignalType=auto
  V/a : Product  Inputs=*/  Multiplication=Element-wise(.*)  SaturateOnIntegerOverflow=on
  Vector norm : aerosimlib/Math/Vector norm
  v/Va : Product  Inputs=*/  Multiplication=Element-wise(.*)  SaturateOnIntegerOverflow=on
  w/u : Product  Inputs=*/  Multiplication=Element-wise(.*)  SaturateOnIntegerOverflow=on
  WindAxesVel : Outport  Port=1
  AlphaBetaDot : Outport  Port=2
  Mach : Outport  Port=3
  wires:
  AOA Saturation/1 -> Mux/3
  Sideslip Saturation/1 -> Mux/2
  Airspeed Saturation/1 -> Mux/1
  V/a/1 -> Mach/1
  SoundSpd/1 -> V/a/2
  Derivative/1 -> AlphaBetaDot/1
  Mux1/1 -> Derivative/1
  Vbody/1 -> Sum/1
  Wbody/1 -> Sum/2
  Sum/1 -> Demux/1, Vector norm/1
  Demux/1 -> w/u/2
  Demux/2 -> v/Va/1
  Demux/3 -> w/u/1
  Vector norm/1 -> Airspeed Saturation/1, v/Va/2, V/a/1
  w/u/1 -> Trigonometric Function/1
  Trigonometric Function/1 -> AOA Saturation/1, Mux1/1
  v/Va/1 -> Trigonometric Function1/1
  Trigonometric Function1/1 -> Sideslip Saturation/1, Mux1/2
  Mux/1 -> WindAxesVel/1

== system tp333079/Aerodynamics/Yaw Moment Coefficient ==
  note: Sources
  note: Rol moment component build-up
  WindAxesVel : Inport  Port=1  PortDimensions=[3 1]  SampleTime=-1  DataType=auto
      settings: SignalType=auto
  Control : Inport  Port=2  PortDimensions=[4 1]  SampleTime=-1  DataType=auto
      settings: SignalType=auto
  AngularRates : Inport  Port=3  PortDimensions=[3 1]  SampleTime=-1  DataType=auto
      settings: SignalType=auto
  2 : Gain  Gain=2  Multiplication=Element-wise(K.*u)  SaturateOnIntegerOverflow=on
  Cn*b/(2V) : Product  Inputs=**/  Multiplication=Element-wise(.*)  SaturateOnIntegerOverflow=on
  Cnbeta : Gain  Gain=Cnbeta  Multiplication=Element-wise(K.*u)  SaturateOnIntegerOverflow=on
  Cnda : Gain  Gain=Cnda  Multiplication=Element-wise(K.*u)  SaturateOnIntegerOverflow=on
  Cndr : Gain  Gain=Cndr  Multiplication=Element-wise(K.*u)  SaturateOnIntegerOverflow=on
  Cnp : Gain  Gain=Cnp  Multiplication=Element-wise(K.*u)  SaturateOnIntegerOverflow=on
  Cnr : Gain  Gain=Cnr  Multiplication=Element-wise(K.*u)  SaturateOnIntegerOverflow=on
  Demux : Demux  Outputs=4  BusSelectionMode=off
  Demux1 : Demux  Outputs=3  BusSelectionMode=off
  Demux3 : Demux  Outputs=3  BusSelectionMode=off
  Sum : Sum  Inputs=++  SaturateOnIntegerOverflow=on
  Sum2 : Sum  Inputs=++++  SaturateOnIntegerOverflow=on
  Terminator{,1..3} (4 alike) : Terminator
  Wing span : Constant  Value=b
  Cn : Outport  Port=1
  wires:
  Cnp/1 -> Sum/1
  Cnr/1 -> Sum/2
  Sum/1 -> Cn*b/(2V)/1
  Wing span/1 -> Cn*b/(2V)/2
  2/1 -> Cn*b/(2V)/3
  WindAxesVel/1 -> Demux1/1
  Demux1/1 -> 2/1
  Demux1/2 -> Cnbeta/1
  Demux1/3 -> Terminator/1
  Demux/1 -> Terminator1/1
  Demux/2 -> Terminator2/1
  Demux/3 -> Cnda/1
  Demux/4 -> Cndr/1
  Control/1 -> Demux/1
  AngularRates/1 -> Demux3/1
  Demux3/1 -> Cnp/1
  Demux3/2 -> Terminator3/1
  Demux3/3 -> Cnr/1
  Cnbeta/1 -> Sum2/1
  Cnda/1 -> Sum2/2
  Cndr/1 -> Sum2/3
  Cn*b/(2V)/1 -> Sum2/4
  Sum2/1 -> Cn/1

== system tp333079/Atmosphere/Background Wind ==
  note: Wind speed in body axes
  WindsNED : Inport  Port=1  PortDimensions=[3 1]  SampleTime=-1  DataType=auto
      settings: SignalType=auto
  DCM : Inport  Port=2  PortDimensions=[3 3]  SampleTime=-1  DataType=auto
      settings: SignalType=auto
  Derivative : Derivative
  Product : Product  Inputs=2  Multiplication=Matrix(*)  SaturateOnIntegerOverflow=on
  Product1 : Product  Inputs=2  Multiplication=Matrix(*)  SaturateOnIntegerOverflow=on
  WindVel : Outport  Port=1
  WindAcc : Outport  Port=2
  wires:
  Product1/1 -> WindAcc/1
  Derivative/1 -> Product1/2
  Product/1 -> WindVel/1
  WindsNED/1 -> Derivative/1, Product/2
  DCM/1 -> Product1/1, Product/1

== system tp333079/Atmosphere/Standard Atmosphere ==
  note: 1976 Standard Atmosphere Look-up Tables
  note: Outputs
  note: Sources
  MSLAlt : Inport  Port=1  PortDimensions=1  SampleTime=-1  DataType=auto
      settings: SignalType=auto
  Density LUT : Lookup  InputValues=stdatm(:,1)  OutputValues=stdatm(:,4)
  Pressure LUT : Lookup  InputValues=stdatm(:,1)  OutputValues=stdatm(:,3)
  Saturation : Saturate  UpperLimit=86000  LowerLimit=0  LinearizeAsGain=on
  Speed of sound  LUT : Lookup  InputValues=stdatm(:,1)  OutputValues=stdatm(:,5)
  Temperature LUT : Lookup  InputValues=stdatm(:,1)  OutputValues=stdatm(:,2)
  p : Outport  Port=1
  T : Outport  Port=2
  rho : Outport  Port=3
  a : Outport  Port=4
  wires:
  Saturation/1 -> Speed of sound  LUT/1, Density LUT/1, Pressure LUT/1, Temperature LUT/1
  Speed of sound  LUT/1 -> a/1
  Density LUT/1 -> rho/1
  Pressure LUT/1 -> p/1
  Temperature LUT/1 -> T/1
  MSLAlt/1 -> Saturation/1

== system tp333079/Atmosphere/Turbulence ==
  note: Sources
  note: Compute turbulence velocity and acceleration
  note: Outputs
  VelW : Inport  Port=1  PortDimensions=[3 1]  SampleTime=-1  DataType=auto
      settings: SignalType=auto
  AGLAlt : Inport  Port=2  PortDimensions=1  SampleTime=-1  DataType=auto
      settings: SignalType=auto
  WindVel : Inport  Port=3  PortDimensions=[3 1]  SampleTime=-1  DataType=auto
      settings: SignalType=auto
  Demux1 : Demux  Outputs=3  BusSelectionMode=off
  Lateral  Turbulence Filter : Subsystem  SimViewingDevice=off  mask(Lateral turbulence filter){tsamp=tsamp}
      mask prompts: tsamp "Sample time [s]:"
      mask help: Shaping filter for lateral turbulence, using von Karman model.
      settings: Permissions=ReadWrite  RTWFcnNameOpts=Auto  RTWFileNameOpts=Auto
  Longitudinal  Turbulence Filter : Subsystem  SimViewingDevice=off  mask(Longitudinal turbulence filter){tsamp=tsamp}
      mask prompts: tsamp "Sample time [s]:"
      mask help: Shaping filter for longitudinal turbulence, using von Karman model.
      settings: Permissions=ReadWrite  RTWFcnNameOpts=Auto  RTWFileNameOpts=Auto
  Mux : Mux  Inputs=3
  Mux1 : Mux  Inputs=3
  Terminator : Terminator
  Terminator1 : Terminator
  Turbulence Characteristics : Subsystem  SimViewingDevice=off
      settings: Permissions=ReadWrite  RTWFcnNameOpts=Auto  RTWFileNameOpts=Auto
      mask Type: Turbulence characteristics
      mask Description: Computes turbulence intensity and reference length as functions of altitude and background wind speed.
  Unit Delay : UnitDelay  X0=0.1  SampleTime=tsamp
  Vertical  Turbulence Filter : Subsystem  SimViewingDevice=off  mask(Vertical turbulence filter){tsamp=tsamp}
      mask prompts: tsamp "Sample time [s]:"
      mask help: Shaping filter for vertical turbulence, using von Karman model.
      settings: Permissions=ReadWrite  RTWFcnNameOpts=Auto  RTWFileNameOpts=Auto
  ft 2 m : aerosimlib/Unit Conversion/Distance/ft 2 m
  ft 2 m1 : aerosimlib/Unit Conversion/Distance/ft 2 m
  m 2 ft : aerosimlib/Unit Conversion/Distance/m 2 ft
  m 2 ft1 : aerosimlib/Unit Conversion/Distance/m 2 ft
  m 2 ft2 : aerosimlib/Unit Conversion/Distance/m 2 ft
  TurbVel : Outport  Port=1
  TurbAcc : Outport  Port=2
  wires:
  Demux1/1 -> m 2 ft/1
  VelW/1 -> Unit Delay/1
  AGLAlt/1 -> m 2 ft1/1
  m 2 ft/1 -> Lateral  Turbulence Filter/1(Airspeed), Vertical  Turbulence Filter/1(Airspeed), Longitudinal  Turbulence Filter/1(Airspeed)
  m 2 ft1/1 -> Turbulence Characteristics/1(AGLAlt)
  WindVel/1 -> m 2 ft2/1
  m 2 ft2/1 -> Turbulence Characteristics/2(WindVel)
  Turbulence Characteristics/1(sigmau) -> Longitudinal  Turbulence Filter/3(Intensity)
  Turbulence Characteristics/2(sigmav) -> Lateral  Turbulence Filter/3(Intensity)
  Turbulence Characteristics/3(sigmaw) -> Vertical  Turbulence Filter/3(Intensity)
  Turbulence Characteristics/4(Lu) -> Longitudinal  Turbulence Filter/2(RefLength)
  Turbulence Characteristics/5(Lv) -> Lateral  Turbulence Filter/2(RefLength)
  Turbulence Characteristics/6(Lw) -> Vertical  Turbulence Filter/2(RefLength)
  Longitudinal  Turbulence Filter/1(LongVel) -> Mux/1
  Longitudinal  Turbulence Filter/2(LongAcc) -> Mux1/1
  Lateral  Turbulence Filter/1(LatVel) -> Mux/2
  Lateral  Turbulence Filter/2(LatAcc) -> Mux1/2
  Vertical  Turbulence Filter/1(VertVel) -> Mux/3
  Vertical  Turbulence Filter/2(VertAcc) -> Mux1/3
  Mux/1 -> ft 2 m/1
  Mux1/1 -> ft 2 m1/1
  ft 2 m/1 -> TurbVel/1
  ft 2 m1/1 -> TurbAcc/1
  Demux1/2 -> Terminator/1
  Demux1/3 -> Terminator1/1
  Unit Delay/1 -> Demux1/1
